simulink model "fast_powertrain"  (R2020b)
settings: Solver=FixedStepAuto  StartTime=0  StopTime=200  RelTol=1e-3
PreLoadFcn:
  | C_sc = 1;
StartFcn:
  | C_sc = 1;
values from neighbouring files (symbols this model uses):
  Ts = old_data.Ts    [model_fc.m]
undefined symbols (not defined in the file or in its folder): DiscIntNeverNeededParam, Ion, Lithium, w
libraries: powerlib x15, lib_converters x3, electricdrivelib x2, fuzblock x1, simulink x1
PostSaveFcn:
  | C_sc = 1;
settings Model: SimulationMode=accelerator  Creator=maloc  LastModifiedBy=maloc
settings DataIOCC: SaveOutput=off  DSMLogging=off
settings OptimizationCC: StrengthReduction=on  PassReuseOutputArgsAs=Individual arguments  LocalBlockOutputs=off  ZeroExternalMemoryAtStartup=off  ZeroInternalMemoryAtStartup=off  OptimizeBlockOrder=speed  OptimizationPriority=Speed  MultiThreadedLoops=on  EfficientTunableParamExpr=on
settings DebuggingCC: RTPrefix=none  StringTruncationChecking=none  AlgebraicLoopMsg=none  ArtificialAlgebraicLoopMsg=none  MaxConsecutiveZCsMsg=none  InheritedTsInSrcMsg=none  MultiTaskDSMMsg=none  MultiTaskCondExecSysMsg=none  MultiTaskRateTransMsg=warning  TasksWithSamePriorityMsg=none  SigSpecEnsureSampleTimeMsg=none  IntegerOverflowMsg=none  Int32ToFloatConvMsg=none  ParameterDowncastMsg=none  ParameterOverflowMsg=none  ParameterPrecisionLossMsg=none  ParameterTunabilityLossMsg=none  FcnCallInpInsideContextMsg=warning  UnconnectedInputMsg=none  UnconnectedOutputMsg=none  UnconnectedLineMsg=none  FrameProcessingCompatibilityMsg=none  BusObjectLabelMismatch=none  RootOutportRequireBusObject=none  UnknownTsInhSupMsg=none  ModelReferenceDataLoggingMessage=none  ModelReferenceExtraNoncontSigs=none  OperatingPointInterfaceChecksumMismatchMsg=none  NonCurrentReleaseOperatingPointMsg=warning  SFUnexpectedBacktrackingDiag=warning  SFNoUnconditionalDefaultTransitionDiag=warning  IntegerSaturationMsg=none
settings SFSimCC: MATLABDynamicMemAlloc=off  SimTargetLang=C++
settings RTWCC: Description=Embedded Coder  SystemTargetFile=ert.tlc  GenCodeOnly=on  TemplateMakefile=ert_default_tmf  GenerateReport=on  BuildConfiguration=Debug  LaunchReport=on
settings CodeAppCC: ForceParamTrailComments=on  IgnoreCustomStorageClasses=off  OperatorAnnotations=on  SimulinkDataObjDesc=on  SFDataObjDesc=on  InsertBlockDesc=on  EnableCustomComments=on
settings ERTTargetCC: TargetLangStandard=C99 (ISO)  GenerateSampleERTMain=on  ERTCustomFileTemplate=example_file_process.tlc

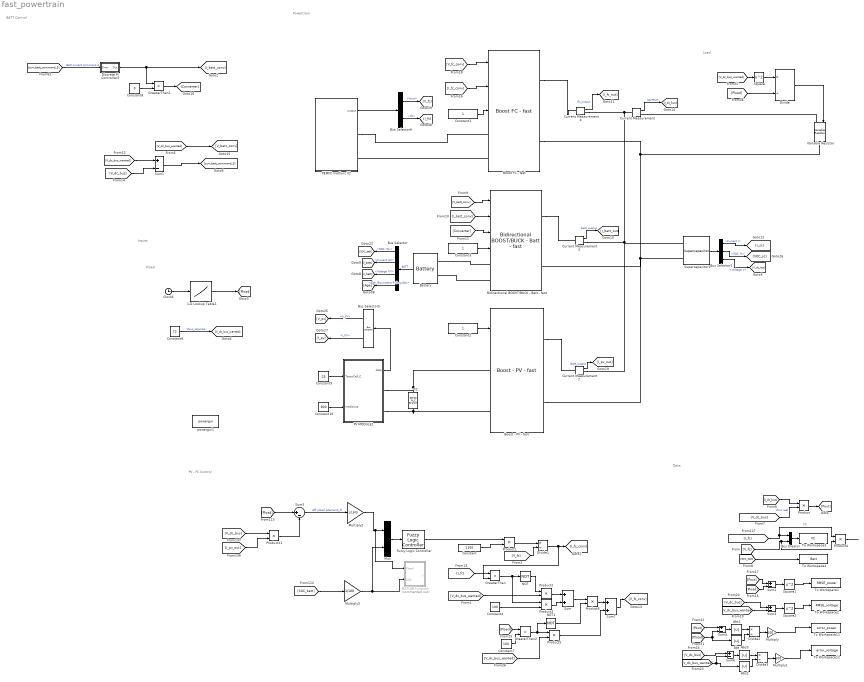
== system fast_powertrain ==
  note: Pload
  note: Data
  note: Powertrain
  note: Load
  note: Inputs
  note: BATT Control
  note: PV - FC Control
  1-D Lookup Table1 : Lookup_n-D  NumberOfTableDimensions=1  BreakpointsForDimension1=t  Table=w  InternalRulePriority=Speed  RndMeth=Simplest  InputSameDT=on
  Abs{,1..3} (4 alike) : Abs
  Battery : electricdrivelib/Extra Sources/Battery  BatType=Lithium-Ion  ShowTempParam=off  ThermalPreset=no  ShowAgeParam=on  NomV=48  NomQ=15  SOC=80  Batt_Tr=20  PresetModel=on  MaxQ=15  MinV=36  FullV=55.8714  Dis_rate=6.5217  R=0.032  Normal_OP=13.5652  expZone="[51.8585     0.736957]"  current=[2 5 10 40]  Units=Time  Tci=20  NomT=20  T2=-30  MaxQ2=4.8  FullV2=7.1  Normal_OP2=5.655  expZone2="[6.58           1]"  Rca=0.6  ti=2000  Dp=0  Neq0=0  Tsim=Ts  Ta1=25  Qeol=5.4*0.9  Reol=0.013333*1.2  Char_age=[2.3478, 3]  Dis_age=[2.3478, 10]  N1=1500  N2=10500  N3=1000  N4=1400  Ta2=45  N5=950
      link override Model/Constant15: Value=Batt_Tr
  Bidirectional BOOST/BUCK - Batt - fast : lib_converters/Bidirectional BOOST//BUCK - Batt - fast  n_buck=0.9  Tr_buck=0.1  damp_buck=0.707  n_boost=0.9  Tr_boost=0.1  damp_boost=0.707  max_curr=[45 -5]  Co=1e-4  CL=C_sc  Li=1e-3  Ts=Ts
  Boost - PV - fast : lib_converters/Boost - PV - fast  n=0.9  Co=1e-4  CL=C_sc  Li=2e-3  damp=0.707  Tr=0.1  Ts=Ts
  Boost FC - fast : lib_converters/Boost FC - fast  conv_type=Average model  n=0.9  Co=1e-4  CL=C_sc  Li=2e-3  damp=0.707  Tr=1  Ts=Ts
  Bus Creator : BusCreator  Inputs=2
  Bus Selector : BusSelector  OutputSignals=SOC (%),Current (A),Voltage (V),Age (Equivalent Full cycles)
  Bus Selector1 : BusSelector  OutputSignals=Current I,SOC %,Voltage V
  Bus Selector5 : BusSelector  OutputSignals=V_PV,I_PV
  Bus Selector6 : BusSelector  OutputSignals=Vout,Ifc
  C2 : powerlib/Elements/Series RLC Branch  LConnTagsString=__new0  RConnTagsString=__new0  BranchType=C  Resistance=0.01  Inductance=1e-3  SetiL0=off  InitialCurrent=0  Capacitance=1e-3  Setx0=off  InitialVoltage=0  Measurements=None
  Clock6 : Clock
  Constant : Constant  Value=1100
  Constant1 : Constant
  Constant10 : Constant  Value=800
  Constant2 : Constant
  Constant3 : Constant
  Constant4 : Constant  Value=100
  Constant6 : Constant  Value=72
  Constant7 : Constant  Value=100
  Constant8 : Constant  Value=0
  Constant9 : Constant  Value=25
  Current Measurement{,2..4} (4 alike) : powerlib/Measurements/Current Measurement  PhasorSimulation=off  OutputType=Complex  PSBequivalent=0
  Discrete PI Controller2 : Subsystem  DialogController=POWERSYS.PowerSysDialog  mask(Discrete PI Controller){Kp=10, Ki=100, Par_Limits=[50 -20], Init=0, Ts=Ts}
      mask prompts: Kp "Proportional gain (Kp):"; Ki "Integral gain (Ki):"; Par_Limits "Output limits: [ Upper   Lower ]"; Init "Output initial value:"; Ts "Sample time:"
      mask help: This block implements a discrete PI controller.
      mask init:
      | UpperLimit=Par_Limits(1);
      | LowerLimit=Par_Limits(2);
      | power_initmask();
      mask Help: This block is part of a subset of blocks in the Extras library that does not have documentation associated with it, other than the block mask description.
      mask Display: disp('PI');
  Divide{,1..3} (4 alike) : Product  Inputs=*/
  Fuzzy Logic Controller : fuzblock/Fuzzy Logic  Controller  FIS='best_sol.fis'  OutputSampleNumber=10  DataType=double  FuzzifiedInputs=off  RuleFiringStrengths=off  RuleOutputs=off  AggregatedOutputs=off  SimulateUsing=Code generation  OutOfRangeInputValueMessage=warning  NoRuleFiredMessage=warning  EmptyOutputFuzzySetMessage=warning
  GreaterThan : RelationalOperator  Operator=<  OutDataTypeStr=boolean  RndMeth=Simplest
  GreaterThan1 : RelationalOperator  Operator=<  OutDataTypeStr=boolean  RndMeth=Simplest
  GreaterThan2 : RelationalOperator  Operator=<  OutDataTypeStr=boolean  RndMeth=Simplest
  MATLAB Function : MATLAB Function  Commented=on  TreatAsAtomicUnit=on
  Multiply : Gain  Gain=100
  Multiply1 : Gain  Gain=100
  Multiply2 : Gain  Gain=1/1500
  Multiply3 : Gain  Gain=1/100
  Mux : Mux  Inputs=2
  NOT : Logic  Operator=NOT  IconShape=distinctive  AllPortsSameDT=off  OutDataTypeStr=boolean
  NOT1 : Logic  Operator=NOT  IconShape=distinctive  AllPortsSameDT=off  OutDataTypeStr=boolean
  PEMFC matfunc V2 : Subsystem  mask{P_H2=0.5, P_O2=1, T=313.15, W=14, tm=1.27e-4, Nfc=50, Rohm=0.061871, Ts=Ts, fc_tau=2}
      mask prompts: P_H2 "Hydrogen pressure (atm)"; P_O2 "Oxygen pressure (atm)"; T "Temperature (K)"; W "Water Content"; tm "Thickness of the membrane (m)"; Nfc "Number of cells"; Rohm "Fuel cell resistance"; Ts "Sample time (s)"; fc_tau "Dynamic response of the FC (s)"
      mask init:
      | tau = fc_tau / 5;
  PV MODULE1 : Subsystem  mask{Npar=1, Nser=1, Ncell=72, Pm=0, Voc=44.5, Isc=5.54, Vmpp=37.2, Impp=4.97, beta_Voc_pc=-0.34, alpha_Isc_pc=-0.017, beta_Voc=0, alpha_Isc=0, IL=5.55564, I0=2.39143e-10, df=0.96618, Rsh=113.762, Rs=0.32122, Ts=Ts}
      mask prompts: Npar "Parallel connected modules"; Nser "Series connected modules"; Ncell "Number of cells per module"; Pm "Maxium Power (W)"; Voc "Open circuit voltage Voc (V)"; Isc "Short-circuit current Isc (A)"; Vmpp "Voltage at MPP (V)"; Impp "Current at MPP (A)"; beta_Voc_pc "Temperature coefficient of Voc (%/deg.C"; alpha_Isc_pc "Temperature coefficient of Isc (%/deg.C)"; beta_Voc "Temperature coefficient of Voc (V/deg.C)"; alpha_Isc "Temperature coefficient of Isc (A/deg.C)"; IL "Light-generated current IL (A)"; I0 "Diode saturation current I0 (A)"; df "Diode ideality factor"; Rsh "Shunt resistance Rsh (ohms)"; Rs "Series resistance Rs (ohms)"; Ts "Sample time (s)"
      mask init:
      | if alpha_Isc ~= 0
      |     alpha = alpha_Isc;
      | else 
      |     alpha = alpha_Isc_pc * Isc/100;
      | end
      mask DialogControl Container5 Prompt: Module data
      mask DialogControl Container3 Prompt: Data from data sheet
      mask DialogControl Container6 Prompt: Data from NREL
  Product{,1..6,21} (8 alike) : Product
  Square : Math  Operator=square  SaturateOnIntegerOverflow=on
  Square1 : Math  Operator=square  SaturateOnIntegerOverflow=on
  Square2 : Math  Operator=square  SaturateOnIntegerOverflow=on
  Sum : Sum
  Sum{1..4,6} (5 alike) : Sum  Inputs=+-
  Sum5 : Sum  Inputs=|+-
  Sum7 : Sum
  Supercapacitor1 : electricdrivelib/Extra Sources/Supercapacitor  C=C_sc  Rdc=150e-3  Voltage=72  Ns=50  Np=1  Vinit=72  Temp=25  PresetModel=on  EstParam=off  Nc=1  r=1e-9  epsilon=6.0208e-10  Ich=10  Vstern="[0.161  2.7  7.8]"  Self_dis=on  Ioc=10  Vself="[48  47.8  47.06  44.65]"  demandeplot=off  I="[10  20 100  500]"  Units=sec  Vmax=0  If=0  deltaV=0.3  alpha=0.3  sec=0
      settings: SourceProductBaseCode=PS
  To Workspace1 : ToWorkspace  VariableName=RMSE_power  SaveFormat=Timeseries  SampleTime=-1
  To Workspace11 : ToWorkspace  VariableName=error_power  SaveFormat=Timeseries  SampleTime=-1
  To Workspace12 : ToWorkspace  VariableName=error_voltage  SaveFormat=Timeseries  SampleTime=-1
  To Workspace2 : ToWorkspace  VariableName=RMSE_voltage  SaveFormat=Timeseries  SampleTime=-1
  To Workspace3 : ToWorkspace  VariableName=FC  SaveFormat=Structure  SampleTime=-1
      settings: Save2DSignal=2-D array (concatenate along first dimension)
  To Workspace4 : ToWorkspace  VariableName=Batt  SaveFormat=Structure  SampleTime=-1
      settings: Save2DSignal=2-D array (concatenate along first dimension)
  Variable Resistor : powerlib/Elements/Variable Resistor  Rabsmin=1e-3
      settings: SourceProductBaseCode=PS
  powergui1 : powerlib/powergui  Priority=1  SimulationMode=Discrete  SampleTime=Ts  frequency=60  Iterations=50  frequencyindice=0  Pbase=100e6  ErrMax=1e-4  UnitsV=kV  UnitsW=MW  buscounter=0  FunctionMessages=off  echomessages=off  EnableUseOfTLC=off  CurrentSourceSwitches=off  DisableSnubberDevices=off  DisableRonSwitches=off  DisableVfSwitches=off  DisplayEquations=off  AutomaticDiscreteSolvers=off  SolverType=Tustin/Backward Euler (TBE)  Interpol=off  ExternalGateDelay=off  methode=off  Ts=100  x0status=blocks  SPID=on  SwTol=0  HookPort=off  NonlinearTolerance=1e-4  nMaxIteration=100  ContinueOnMaxIteration=off  RestoreLinks=warning  ResistiveCurrentMeasurement=off  Frange=[0:2:500]  Ylog=off  Xlog=on  ShowGrid=off  save=off  variable=ZData  structure=0  ZoomFFT=off  StartTime=0.0  cycles=1  DisplayStyle=1  fundamental=60  FreqAxis=off  MaxFrequency=1000  frequencyindicesteady=1  RmsSteady=1  display=off
  wires:
  Constant6/1 -> [V_dc_bus_wanted]  "Vbus_required"
  Battery/1 -> Bus Selector/1  "BATT"
  Current Measurement4/1 -> [I_fc_out]  "Ifc_output"
  Current Measurement3/1 -> [I_batt_out]  "Ibatt_output"
  Supercapacitor1/1 -> Bus Selector1/1
  Bus Selector/3 -> [V_batt]  "<Voltage (V)>"
  Bus Selector1/1 -> [I_sc]  "<Current I>"
  Current Measurement/1 -> [I_dc_bus]  "OUTPUT"
  Current Measurement2/1 -> [I_pv_out]  "Ibatt_output"
  Bus Selector/1 -> [SOC_batt]  "<SOC (%)>"
  [V_dc_bus_wanted] -> Square/1
  Square/1 -> Divide/1
  [Pload] -> Divide/2
  Divide/1 -> Variable Resistor/1
  Bus Selector1/2 -> [SOC_sc]  "<SOC %>"
  [I_fc] -> Product4/1, Bus Creator/1  "FC"
  Clock6/1 -> 1-D Lookup Table1/1
  1-D Lookup Table1/1 -> [Pload]
  Constant9/1 -> PV MODULE1/1(TempCell_C)
  Constant10/1 -> PV MODULE1/2(Irradiance)
  PV MODULE1/1(data) -> Bus Selector5/1
  Bus Selector/4 -> [Age]  "<Age (Equivalent Full cycles)>"
  PEMFC matfunc V2/1(output) -> Bus Selector6/1
  Bus Selector6/1 -> [V_fc]  "<Vout>"
  Bus Selector6/2 -> [I_fc]  "<Ifc>"
  [SOC_batt] -> Multiply3/1
  [V_dc_bus] -> Product21/1
  [curr_batt_command_3] -> Discrete PI Controller2/1(Error)  "Batt current command 3"
  [V_dc_bus_wanted] -> [V_batt_conv]
  [Pload] -> Sum5/1
  Product21/1 -> Sum5/2
  Mux/1 -> Fuzzy Logic Controller/1
  [I_pv_out] -> Product21/2
  Sum5/1 -> Multiply2/1  "diff pload pdemand_fc"
  Bus Selector1/3 -> [V_dc_bus]  "<Voltage V>"
  Product/1 -> [Pout]
  [I_dc_bus] -> Product/1
  [V_dc_bus] -> Product/2  "Vbus real"
  [SOC_batt] -> To Workspace4/1
  [Converter] -> Bidirectional BOOST/BUCK - Batt - fast/3
  [I_batt_conv] -> Bidirectional BOOST/BUCK - Batt - fast/2
  [V_batt_conv] -> Bidirectional BOOST/BUCK - Batt - fast/1
  Constant3/1 -> Bidirectional BOOST/BUCK - Batt - fast/4
  Constant2/1 -> Boost - PV - fast/1
  Constant1/1 -> Boost FC - fast/3
  [I_fc_conv] -> Boost FC - fast/2
  [V_fc_conv] -> Boost FC - fast/1
  Product1/1 -> Divide1/1
  Constant/1 -> Product1/2
  [V_fc] -> Divide1/2
  Divide1/1 -> GreaterThan/2, [I_fc_conv]
  [I_fc] -> GreaterThan/1
  GreaterThan/1 -> NOT/1, Product3/1
  Product2/1 -> Sum/1
  [V_dc_bus_wanted] -> Product2/2
  Sum7/1 -> [V_fc_conv]
  Product3/1 -> Sum/2
  Constant4/1 -> Product3/2
  NOT/1 -> Product2/1
  [V_dc_bus_wanted] -> Sum1/1
  [V_dc_bus] -> Sum1/2
  Sum1/1 -> [curr_batt_command_3]
  GreaterThan1/1 -> [Converter]
  Constant8/1 -> GreaterThan1/2
  Sum2/1 -> Square1/1
  [V_dc_bus] -> Sum3/1
  [Pout] -> Sum2/1
  [Pload] -> Sum2/2
  Sum3/1 -> Square2/1
  [V_dc_bus_wanted] -> Sum3/2
  Sum4/1 -> Abs1/1
  Abs1/1 -> Divide2/1
  Abs/1 -> Divide2/2
  Divide2/1 -> Multiply/1
  [Pload] -> Abs/1, Sum4/2
  [Pout] -> Sum4/1
  [V_dc_bus] -> Sum6/1
  [V_dc_bus_wanted] -> Abs2/1, Sum6/2
  Divide3/1 -> Multiply1/1
  Abs2/1 -> Divide3/2
  Abs3/1 -> Divide3/1
  Sum6/1 -> Abs3/1
  Square1/1 -> To Workspace1/1
  Square2/1 -> To Workspace2/1
  Multiply/1 -> To Workspace11/1
  Multiply1/1 -> To Workspace12/1
  Bus Creator/1 -> To Workspace3/1
  [V_fc] -> Product4/2, Bus Creator/2
  Bus Selector/2 -> [I_batt]  "<Current (A)>"
  Bus Selector5/2 -> [I_pv]  "<I_PV>"
  Discrete PI Controller2/1(Out) -> [I_batt_conv], GreaterThan1/1
  Bus Selector5/1 -> [V_pv]  "<V_PV>"
  [Pload] -> GreaterThan2/1
  Constant7/1 -> GreaterThan2/2
  GreaterThan2/1 -> NOT1/1, Product5/1
  [V_dc_bus_wanted] -> Product5/2
  NOT1/1 -> Product6/2
  Sum/1 -> Product6/1
  Product6/1 -> Sum7/1
  Product5/1 -> Sum7/2
  Product4/1 -> ?
  Multiply2/1 -> MATLAB Function/1(Pload), Mux/1
  Multiply3/1 -> Mux/2, MATLAB Function/2(SOC)
  Fuzzy Logic Controller/1 -> Product1/1
  connections:
  Variable Resistor/LConn1 -- Current Measurement/RConn1
  Variable Resistor/RConn1 -- Boost - PV - fast/RConn2 -- Bidirectional BOOST/BUCK - Batt - fast/RConn2 -- Supercapacitor1/LConn2 -- Boost FC - fast/RConn2
  Current Measurement/LConn1 -- Current Measurement4/RConn1 -- Supercapacitor1/LConn1 -- Current Measurement2/RConn1 -- Current Measurement3/RConn1
  Bidirectional BOOST/BUCK - Batt - fast/LConn2 -- Battery/LConn2
  Bidirectional BOOST/BUCK - Batt - fast/LConn1 -- Battery/LConn1
  Bidirectional BOOST/BUCK - Batt - fast/RConn1 -- Current Measurement3/LConn1
  Boost FC - fast/RConn1 -- Current Measurement4/LConn1
  C2/RConn1 -- Boost - PV - fast/LConn2 -- PV MODULE1/RConn2
  Boost - PV - fast/RConn1 -- Current Measurement2/LConn1
  PV MODULE1/RConn1 -- C2/LConn1 -- Boost - PV - fast/LConn1
  PEMFC matfunc V2/RConn1 -- Boost FC - fast/LConn1
  Boost FC - fast/LConn2 -- PEMFC matfunc V2/RConn2

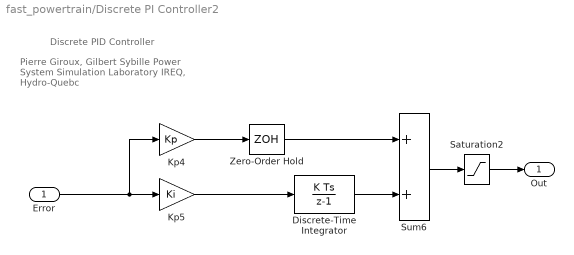
== system fast_powertrain/Discrete PI Controller2 ==
  note: Pierre Giroux, Gilbert Sybille
      | Power System Simulation Laboratory
      | IREQ, Hydro-Quebc
  note: Discrete PID Controller
  Error : Inport  SampleTime=Ts
  Discrete-Time Integrator : DiscreteIntegrator  InitialCondition=Init  SampleTime=Ts  LimitOutput=on  UpperSaturationLimit=UpperLimit  LowerSaturationLimit=LowerLimit  ICPrevOutput=DiscIntNeverNeededParam  ICPrevScaledInput=DiscIntNeverNeededParam
  Kp4 : Gain  Gain=Kp  SaturateOnIntegerOverflow=on  SampleTime=Ts  OutDataTypeStr=Inherit: Same as input  ParamDataTypeStr=Inherit: Same as input
  Kp5 : Gain  Gain=Ki  SaturateOnIntegerOverflow=on  SampleTime=Ts  OutDataTypeStr=Inherit: Same as input  ParamDataTypeStr=Inherit: Same as input
  Saturation2 : Saturate  UpperLimit=UpperLimit  LowerLimit=LowerLimit  SampleTime=Ts
  Sum6 : Sum  InputSameDT=on  SaturateOnIntegerOverflow=on  SampleTime=Ts  OutDataTypeStr=Inherit: Same as first input
  Zero-Order Hold : ZeroOrderHold  SampleTime=Ts
  Out : Outport  SampleTime=Ts  InitialOutput=0  VectorParamsAs1DForOutWhenUnconnected=off
  wires:
  Error/1 -> Kp4/1, Kp5/1
  Sum6/1 -> Saturation2/1
  Kp5/1 -> Discrete-Time Integrator/1
  Kp4/1 -> Zero-Order Hold/1
  Discrete-Time Integrator/1 -> Sum6/2
  Saturation2/1 -> Out/1
  Zero-Order Hold/1 -> Sum6/1

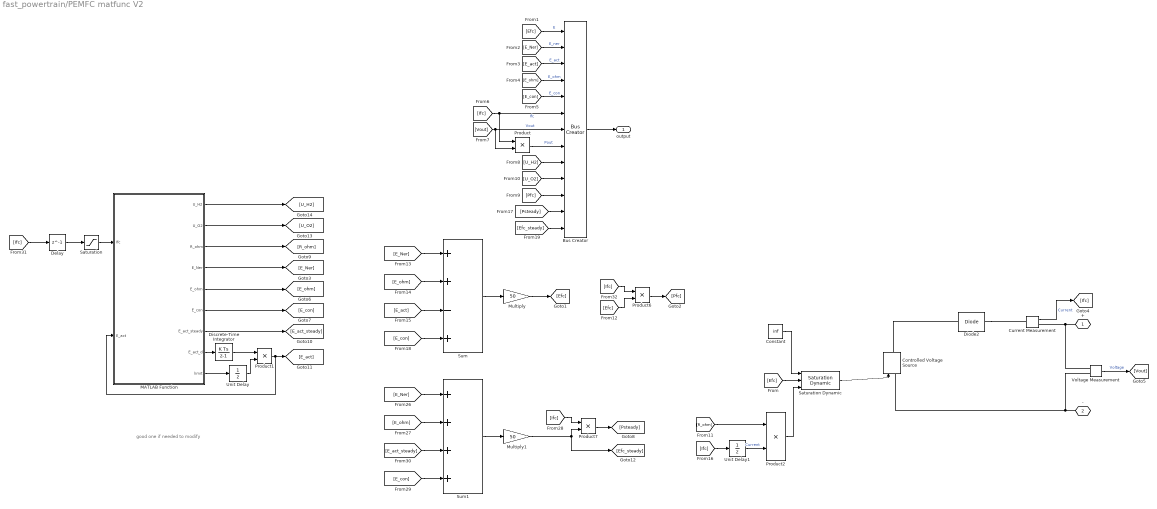
== system fast_powertrain/PEMFC matfunc V2 ==
  note: good one if needed to modify
  Bus Creator : BusCreator  Inputs=13
  Constant : Constant  Value=inf
  Controlled Voltage Source : powerlib/Electrical Sources/Controlled Voltage Source  Initialize=on  Source_Type=AC  Amplitude=0  Phase=0  Frequency=0  Measurements=None
  Current Measurement : powerlib/Measurements/Current Measurement  PhasorSimulation=off  OutputType=Complex  PSBequivalent=0
  Delay : Delay  DelayLength=1
  Diode2 : powerlib/Power Electronics/Diode  Ron=Rohm  Lon=0  Vf=0  IC=0  UseSnubber=off  Rs=1e4  Cs=inf  Measurements=off
  Discrete-Time Integrator : DiscreteIntegrator  SampleTime=-1  ICPrevOutput=DiscIntNeverNeededParam  ICPrevScaledInput=DiscIntNeverNeededParam
  MATLAB Function : MATLAB Function  TreatAsAtomicUnit=on
  Multiply : Gain  Gain=50
  Multiply1 : Gain  Gain=50
  Product{,1..2,6..7} (5 alike) : Product
  Saturation : Saturate  UpperLimit=inf  LowerLimit=0.001
  Saturation Dynamic : simulink/Discontinuities/Saturation Dynamic  OutMin=[]  OutMax=[]  OutDataTypeStr=Inherit: Same as second input  OutDataType=fixdt(1, 16)  OutScaling=2^-10  DoSatur=off
  Sum : Sum  Inputs=++-+
  Sum1 : Sum  Inputs=++++
  Unit Delay : UnitDelay  SampleTime=-1  HasFrameUpgradeWarning=on
  Unit Delay1 : UnitDelay  SampleTime=Ts  HasFrameUpgradeWarning=on
  Voltage Measurement : powerlib/Measurements/Voltage Measurement  PhasorSimulation=off  OutputType=Complex  PSBequivalent=0
  + : PMIOPort  Tag=PMCPort  Side=Right
  - : PMIOPort  Tag=PMCPort  Port=2  Side=Right
  output : Outport  VectorParamsAs1DForOutWhenUnconnected=off
  wires:
  [Efc] -> Bus Creator/1  "E"
  [E_Ner] -> Bus Creator/2  "E_ner"
  [E_act] -> Bus Creator/3  "E_act"
  [E_ohm] -> Bus Creator/4  "E_ohm"
  [Ifc] -> Product/1, Bus Creator/6  "Ifc"
  [Vout] -> Product/2, Bus Creator/7  "Vout"
  [E_con] -> Bus Creator/5  "E_con"
  Product/1 -> Bus Creator/8  "Pout"
  Current Measurement/1 -> [Ifc]  "Current"
  Voltage Measurement/1 -> [Vout]  "Voltage"
  [U_H2] -> Bus Creator/9
  [U_O2] -> Bus Creator/10
  Bus Creator/1 -> output/1
  [Ifc] -> Unit Delay1/1
  Unit Delay1/1 -> Product2/2  "Current"
  Product2/1 -> Saturation Dynamic/3
  [R_ohm] -> Product2/1
  Constant/1 -> Saturation Dynamic/1
  Saturation Dynamic/1 -> Controlled Voltage Source/1
  MATLAB Function/3(R_ohm) -> [R_ohm]
  MATLAB Function/7(E_act_steady) -> [E_act_steady]
  MATLAB Function/5(E_ohm) -> [E_ohm]
  Discrete-Time Integrator/1 -> Product1/1
  [Efc] -> Product6/2
  [E_ohm] -> Sum1/2
  Multiply1/1 -> [Efc_steady], Product7/2
  [E_con] -> Sum1/4
  [Ifc] -> Product7/1
  [E_ohm] -> Sum/2
  [E_act] -> Sum/3
  Product6/1 -> [Pfc]
  [E_act_steady] -> Sum1/3
  Sum1/1 -> Multiply1/1
  Sum/1 -> Multiply/1
  MATLAB Function/4(E_Ner) -> [E_Ner]
  [E_con] -> Sum/4
  MATLAB Function/6(E_con) -> [E_con]
  [Ifc] -> Product6/1
  [E_Ner] -> Sum1/1
  [Ifc] -> Delay/1
  Multiply/1 -> [Efc]
  MATLAB Function/8(E_act_d) -> Discrete-Time Integrator/1
  [E_Ner] -> Sum/1
  [Efc] -> Saturation Dynamic/2
  Product7/1 -> [Psteady]
  [Efc_steady] -> Bus Creator/13
  [Pfc] -> Bus Creator/11
  [Psteady] -> Bus Creator/12
  MATLAB Function/1(U_H2) -> [U_H2]
  MATLAB Function/2(U_O2) -> [U_O2]
  Saturation/1 -> MATLAB Function/1(Ifc)
  Delay/1 -> Saturation/1
  Product1/1 -> MATLAB Function/2(E_act), [E_act]
  MATLAB Function/9(limit) -> Unit Delay/1
  Unit Delay/1 -> Product1/2
  connections:
  -/RConn1 -- Voltage Measurement/LConn2 -- Controlled Voltage Source/LConn1
  +/RConn1 -- Voltage Measurement/LConn1 -- Current Measurement/RConn1
  Diode2/RConn1 -- Current Measurement/LConn1
  Diode2/LConn1 -- Controlled Voltage Source/RConn1

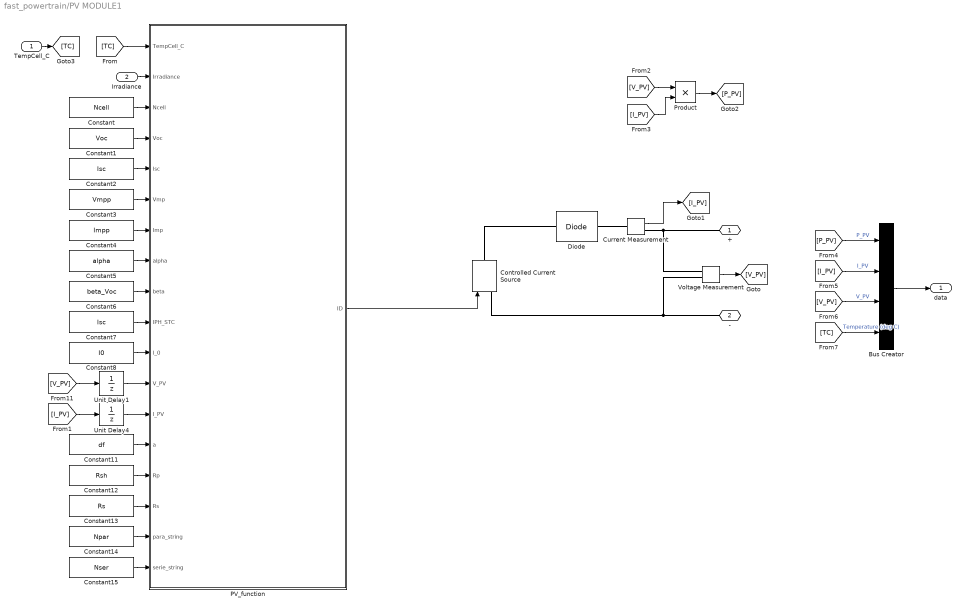
== system fast_powertrain/PV MODULE1 ==
  TempCell_C : Inport
  Irradiance : Inport  Port=2
  Bus Creator : BusCreator  Inputs=4
  Constant : Constant  Value=Ncell
  Constant1 : Constant  Value=Voc
  Constant11 : Constant  Value=df
  Constant12 : Constant  Value=Rsh
  Constant13 : Constant  Value=Rs
  Constant14 : Constant  Value=Npar
  Constant15 : Constant  Value=Nser
  Constant2 : Constant  Value=Isc
  Constant3 : Constant  Value=Vmpp
  Constant4 : Constant  Value=Impp
  Constant5 : Constant  Value=alpha
  Constant6 : Constant  Value=beta_Voc
  Constant7 : Constant  Value=Isc
  Constant8 : Constant  Value=I0
  Controlled Current Source : powerlib/Electrical Sources/Controlled Current Source  Initialize=on  Source_Type=AC  Amplitude=0  Phase=0  Frequency=0  Measurements=None
  Current Measurement : powerlib/Measurements/Current Measurement  PhasorSimulation=off  OutputType=Complex  PSBequivalent=0
  Diode : powerlib/Power Electronics/Diode  Ron=0.001  Lon=0  Vf=0.8  IC=0  UseSnubber=0  Rs=500  Cs=250e-9  Measurements=off
  PV_function : MATLAB Function  TreatAsAtomicUnit=on
  Product : Product
  Unit Delay1 : UnitDelay  SampleTime=Ts  HasFrameUpgradeWarning=on
  Unit Delay4 : UnitDelay  SampleTime=Ts  HasFrameUpgradeWarning=on
  Voltage Measurement : powerlib/Measurements/Voltage Measurement  PhasorSimulation=off  OutputType=Complex  PSBequivalent=0
  + : PMIOPort  Side=Right
  - : PMIOPort  Port=2  Side=Right
  data : Outport
  wires:
  [V_PV] -> Unit Delay1/1
  [I_PV] -> Unit Delay4/1
  Unit Delay4/1 -> PV_function/13(I_PV)
  Unit Delay1/1 -> PV_function/12(V_PV)
  Bus Creator/1 -> data/1
  [V_PV] -> Bus Creator/3  "V_PV"
  [I_PV] -> Bus Creator/2  "I_PV"
  [P_PV] -> Bus Creator/1  "P_PV"
  Product/1 -> [P_PV]
  [I_PV] -> Product/2
  [V_PV] -> Product/1
  Current Measurement/1 -> [I_PV]
  Voltage Measurement/1 -> [V_PV]
  Constant12/1 -> PV_function/15(Rp)
  Constant8/1 -> PV_function/11(I_0)
  Constant13/1 -> PV_function/16(Rs)
  Constant11/1 -> PV_function/14(a)
  PV_function/1(ID) -> Controlled Current Source/1
  Constant2/1 -> PV_function/5(Isc)
  Constant4/1 -> PV_function/7(Imp)
  Constant5/1 -> PV_function/8(alpha)
  Constant7/1 -> PV_function/10(IPH_STC)
  TempCell_C/1 -> [TC]
  Constant6/1 -> PV_function/9(beta)
  Constant1/1 -> PV_function/4(Voc)
  Irradiance/1 -> PV_function/2(Irradiance)
  Constant14/1 -> PV_function/17(para_string)
  Constant15/1 -> PV_function/18(serie_string)
  Constant3/1 -> PV_function/6(Vmp)
  Constant/1 -> PV_function/3(Ncell)
  [TC] -> Bus Creator/4  "Temperature (deg C)"
  [TC] -> PV_function/1(TempCell_C)
  connections:
  Diode/LConn1 -- Controlled Current Source/RConn1
  Current Measurement/LConn1 -- Diode/RConn1
  Voltage Measurement/LConn1 -- +/RConn1 -- Current Measurement/RConn1
  Controlled Current Source/LConn1 -- Voltage Measurement/LConn2 -- -/RConn1

== matlab function fast_powertrain/MATLAB Function ==
  settings: updateMethod=DISCRETE  sampleTime=Ts
  data: Pload input; y output; SOC input
function y = fcn(Pload, SOC)
y = 0;
coder.extrinsic('test_fcn');

persistent myfis;
if isempty(myfis)
    myfis = getFISCodeGenerationData('best_sol.fis');
end


% % m = [Pload SOC];
% y = [0];
% m = evalfis(myfis,[0.5 0.5]);
% y = m(1);


y = test_fcn(myfis,Pload, SOC);
% m = evalfis(myfis);
% y = m(1);

== matlab function fast_powertrain/PV MODULE1/PV_function ==
  settings: updateMethod=DISCRETE  sampleTime=Ts
  data: TempCell_C input; ID output; Irradiance input; Ncell input; Voc input; Isc input; Vmp input; Imp input; alpha input; beta input; IPH_STC input; I_0 input; V_PV input; I_PV input; a input; Rp input; Rs input; para_string input; serie_string input
function ID = pv_calculation(TempCell_C, Irradiance, Ncell, Voc, Isc, Vmp, Imp, alpha, beta, IPH_STC, I_0,V_PV, I_PV, a, Rp, Rs, para_string, serie_string)
    %% Constant
    n = a;
    Tc_STC = 25 + 273.15;
    G_STC = 1000;
    TempCell_K = TempCell_C+273.15;
    
    k = 1.3806e-23; % Boltzman constant (J/K)
    k_ = 8.617333262145e-5; % Boltzman constant (eV/K)
    q = 1.602e-19; % Elementary charge on an electron (C)
    % k_ = k/q;
    Eg0 = 1.121;
    Eg_ref = Eg0*q; % Band gap for silicon (eV)
    
    
    

%     
%     if isnan(V_PV)
%         V_PV = 0;
%     end
%     if isnan(I_PV)
%         I_PV = 0;
%     end
    
    
    %% Method 2 + Ncell dans Id + -1 dans Irs + Ish différent
    %     Voc = Voc / Ncell;
    k = 1.3806e-23;
    Vt = k/q*TempCell_K;
    IPH = ((TempCell_K-Tc_STC)*alpha+IPH_STC)*para_string*Irradiance/G_STC;
    Ish = (V_PV + I_PV*Rs)/Rp;
    Irs = IPH_STC/(exp(q*Voc/(Ncell*k*a*TempCell_K))-1);
    Is = Irs * (TempCell_K/Tc_STC)^3*exp((Eg_ref/(k_*a))*(1/TempCell_K - 1/Tc_STC));
    % Maybe change above ? (1/Tc_STC - 1/TempCell_K) ??
    Id = para_string * Is * (exp((V_PV/serie_string+I_PV*Rs/para_string)/(n*Vt*Ncell))-1);
    ID = IPH * para_string - Ish - Id;
    
end


% https://hal.archives-ouvertes.fr/hal-01351308/document
% PV -> autre -> Matlab sim model
% PV -> autre -> PV panel
% PV -> autre -> PV module
% https://environmentalsystemsresearch.springeropen.com/articles/10.1186/s40068-015-0047-9
% https://iopscience.iop.org/article/10.1088/1757-899X/114/1/012137/pdf

== matlab function fast_powertrain/PEMFC matfunc V2/MATLAB Function ==
  settings: updateMethod=DISCRETE  sampleTime=Ts
  data: U_H2 output; U_O2 output; R_ohm output; Ifc input; E_Ner output; E_ohm output; E_con output; E_act_steady output; E_act input; E_act_d output; limit output
function [U_H2,U_O2,R_ohm,E_Ner,E_ohm,E_con,E_act_steady,E_act_d,limit] = fcn(Ifc,E_act)
%     https://link.springer.com/article/10.1007/s40565-016-0196-5
%     Modeling and Simulation of a Proton Exchange Membrane Fuel Cell Alongside a Waste Heat Recovery System Based on the Organic Rankine Cycle in MATLAB/SIMULINK Environment
%     MATHEMATICAL MODELLING FOR PROTON EXCHANGE MEMBRANE FUEL CELL (PEMFC) 
%     https://www.scirp.org/pdf/epe_2020112310053180.pdf#page=17&zoom=100,72,604
%     H-Series Fuel Cell Stacks

    %% constants:
    R = 8.3145;
    Pstd = 101325;
    nF = 2*96485;
    C_act = 2;
    A = 19.6*4.0;
    T = 303.15;
    Nfc = 50;
    lambda = 14;
    l = 21e-4 * 10^-2;
%     l = 1.27e-4;
    
    J = Ifc/A;
    JM = 45/A;
    Pa = 1.45;
    Pc = 1;
    Tc = T-273.15;
    coeff = 1;
        
%     if Ifc <=0
%         Ifc = 40;
%     end
    
    PH2Osat = 10^(-2.18+2.95e-2*Tc-9.18e-5*Tc^2+1.44e-7*Tc^3);
    
    P_H2 = 0.5*PH2Osat*(exp(-(1.635*J/T^1.334))*(Pa/PH2Osat)-1);
    P_O2 = PH2Osat*(exp(-(4.192*J/T^1.334))*(Pc/PH2Osat)-1);
    

    %% Saturation at start
    if -1.87e-4*log(Ifc) > 0
        k = 0;
    else
        if -1.87e-4*log(Ifc) < -1.2
            k = -1.2;
        else
            k = -1.87e-4*log(Ifc);
        end
    end
    %% Nernst Voltage
    E_Ner = 1.229 + (T-298.15) * (-0.85e-3) + T*R/nF * log(P_H2*P_O2^0.5);
    
    %% Activation loss
    % Pressure not in Pa ?
    CO2 = (P_O2/(5.08e6))*exp(498/T);
    CH2 = (P_H2/(1.09e6))*exp(-77/T);
    E_act_steady=-0.9514 + T * (2.86e-3+2e-4*log(200)+4.3e-5*log(CH2)+7.4e-5*log(CO2)+k);
%     E_act_steady = -0.9514 + 3.12e-3*T + 7.4e-5*T*log(CO2) -1.87e-4*T*log(Ifc);
    
    %% Ohmic loss
    E_ohm = - Ifc*(l/((lambda*5.139e-3-3.26e-3)*exp(1268*(1/303-1/T))));
    R_ohm = (l/((lambda*5.139e-3-3.26e-3)*exp(1268*(1/303-1/T))));
    
    %% Concentration loss
%     if T>= 312.15
%         E_con = (1.1e-4-1.2e-6*(T-273.15))*exp(8*Ifc/40);
%     else
%         E_con = (3.3e-3-8.2e-5*(T-273.15))*exp(8*Ifc/40);
%     end

%     E_con = 3*R*T/(2*nF)*log(1-J/JM)-1.5607*R*T/(2*nF);
        if J/JM < 1
        E_con = 3*R*T/(2*nF)*log(1-J/JM)-1.5607*R*T/(2*nF);
    else
%         E_con = -abs(3*R*T/(2*nF)*log(complex(1-J/(JM-0.001)))-1.5607*R*T/(2*nF));
        E_con = 3*R*T/(2*nF)*log(J/JM)-1.5607*R*T/(2*nF);
    end
    
    %% with coefficient
    E_con = coeff * E_con;
    E_act_steady = coeff * E_act_steady;
    E_ohm = coeff * E_ohm;
    E_Ner = coeff * E_Ner;
    
        
    %% activation dynamic loss:
    below = -E_act_steady-E_con;
    E_act_d = (Ifc/C_act)*(1-E_act/below);
%     E_act_d = 0;

    %% Fuel utilization
    U_H2 = 60000*Ifc*R*T*Nfc/(nF*1.16*1*0.9995*Pstd);
    
    %% Air utilization
    U_O2 = 60000*Ifc*R*T*Nfc/(2*nF*0.0181*1*0.21*Pstd);
    limit = 1;
    if J/JM >= 1
            E_con = 0;
            E_act_steady = 0;
            E_ohm = 0;
            E_act_d = 0;
            E_Ner = -35*Ifc;
            if E_Ner <= 0
                E_Ner = 0;
            end
            limit = 0;
    end
end
